simulink model "run_small_function_cov_bitadder"  (R2022b)
settings: Solver=VariableStepAuto  StartTime=0.0  StopTime=0.0  RelTol=1e-3
libraries: simulink x3193, hdlsllib x1590, ece1718_small_function x16
(part 25 of 26)

== system run_small_function_cov_bitadder/For Iterator Subsystem/train_top/batch/train_sub/conv_sig/filter dim iter /i ietar Subsystem/Subsystem/For Iterator Subsystem/mac/wt_multi/ca32/fa25 ==
  in1 : Inport  OutDataTypeStr=fixdt(0, 1, 0)  SampleTime=-1
  in2 : Inport  Port=2  OutDataTypeStr=fixdt(0, 1, 0)  SampleTime=-1
  Cin : Inport  Port=3  OutDataTypeStr=fixdt(0, 1, 0)  SampleTime=-1
  Bit_AND : simulink/Logic and Bit Operations/Bitwise Operator  logicop=AND  UseBitMask=off  NumInputPorts=2  BitMask=double(0)  BitMaskRealWorld=Real World Value
  Bit_AND_1 : simulink/Logic and Bit Operations/Bitwise Operator  logicop=AND  UseBitMask=off  NumInputPorts=2  BitMask=double(0)  BitMaskRealWorld=Real World Value
  Bit_OR : simulink/Logic and Bit Operations/Bitwise Operator  logicop=OR  UseBitMask=off  NumInputPorts=2  BitMask=double(0)  BitMaskRealWorld=Real World Value
  Bit_XOR : simulink/Logic and Bit Operations/Bitwise Operator  logicop=XOR  UseBitMask=off  NumInputPorts=2  BitMask=double(0)  BitMaskRealWorld=Real World Value
  Bit_XOR_1 : simulink/Logic and Bit Operations/Bitwise Operator  logicop=XOR  UseBitMask=off  NumInputPorts=2  BitMask=double(0)  BitMaskRealWorld=Real World Value
  Bit_XOR_2 : simulink/Logic and Bit Operations/Bitwise Operator  logicop=XOR  UseBitMask=off  NumInputPorts=2  BitMask=double(0)  BitMaskRealWorld=Real World Value
  S : Outport  OutDataTypeStr=fixdt(0, 1, 0)  SampleTime=-1
  C : Outport  Port=2  OutDataTypeStr=fixdt(0, 1, 0)  SampleTime=-1
  wires:
  in1/1 -> Bit_XOR_2/1, Bit_AND/1, Bit_XOR_1/1
  Cin/1 -> Bit_AND_1/1, Bit_XOR/2
  Bit_XOR/1 -> S/1
  Bit_AND/1 -> Bit_OR/1
  in2/1 -> Bit_XOR_2/2, Bit_AND/2, Bit_XOR_1/2
  Bit_AND_1/1 -> Bit_OR/2
  Bit_OR/1 -> C/1
  Bit_XOR_2/1 -> Bit_AND_1/2
  Bit_XOR_1/1 -> Bit_XOR/1

== system run_small_function_cov_bitadder/For Iterator Subsystem/train_top/batch/train_sub/conv_sig/filter dim iter /i ietar Subsystem/Subsystem/For Iterator Subsystem/mac/wt_multi/ca32/fa26 ==
  in1 : Inport  OutDataTypeStr=fixdt(0, 1, 0)  SampleTime=-1
  in2 : Inport  Port=2  OutDataTypeStr=fixdt(0, 1, 0)  SampleTime=-1
  Cin : Inport  Port=3  OutDataTypeStr=fixdt(0, 1, 0)  SampleTime=-1
  Bit_AND : simulink/Logic and Bit Operations/Bitwise Operator  logicop=AND  UseBitMask=off  NumInputPorts=2  BitMask=double(0)  BitMaskRealWorld=Real World Value
  Bit_AND_1 : simulink/Logic and Bit Operations/Bitwise Operator  logicop=AND  UseBitMask=off  NumInputPorts=2  BitMask=double(0)  BitMaskRealWorld=Real World Value
  Bit_OR : simulink/Logic and Bit Operations/Bitwise Operator  logicop=OR  UseBitMask=off  NumInputPorts=2  BitMask=double(0)  BitMaskRealWorld=Real World Value
  Bit_XOR : simulink/Logic and Bit Operations/Bitwise Operator  logicop=XOR  UseBitMask=off  NumInputPorts=2  BitMask=double(0)  BitMaskRealWorld=Real World Value
  Bit_XOR_1 : simulink/Logic and Bit Operations/Bitwise Operator  logicop=XOR  UseBitMask=off  NumInputPorts=2  BitMask=double(0)  BitMaskRealWorld=Real World Value
  Bit_XOR_2 : simulink/Logic and Bit Operations/Bitwise Operator  logicop=XOR  UseBitMask=off  NumInputPorts=2  BitMask=double(0)  BitMaskRealWorld=Real World Value
  S : Outport  OutDataTypeStr=fixdt(0, 1, 0)  SampleTime=-1
  C : Outport  Port=2  OutDataTypeStr=fixdt(0, 1, 0)  SampleTime=-1
  wires:
  in1/1 -> Bit_XOR_2/1, Bit_AND/1, Bit_XOR_1/1
  in2/1 -> Bit_XOR_2/2, Bit_AND/2, Bit_XOR_1/2
  Cin/1 -> Bit_AND_1/1, Bit_XOR/2
  Bit_AND_1/1 -> Bit_OR/2
  Bit_OR/1 -> C/1
  Bit_AND/1 -> Bit_OR/1
  Bit_XOR_2/1 -> Bit_AND_1/2
  Bit_XOR/1 -> S/1
  Bit_XOR_1/1 -> Bit_XOR/1

== system run_small_function_cov_bitadder/For Iterator Subsystem/train_top/batch/train_sub/conv_sig/filter dim iter /i ietar Subsystem/Subsystem/For Iterator Subsystem/mac/wt_multi/ca32/fa27 ==
  in1 : Inport  OutDataTypeStr=fixdt(0, 1, 0)  SampleTime=-1
  in2 : Inport  Port=2  OutDataTypeStr=fixdt(0, 1, 0)  SampleTime=-1
  Cin : Inport  Port=3  OutDataTypeStr=fixdt(0, 1, 0)  SampleTime=-1
  Bit_AND : simulink/Logic and Bit Operations/Bitwise Operator  logicop=AND  UseBitMask=off  NumInputPorts=2  BitMask=double(0)  BitMaskRealWorld=Real World Value
  Bit_AND_1 : simulink/Logic and Bit Operations/Bitwise Operator  logicop=AND  UseBitMask=off  NumInputPorts=2  BitMask=double(0)  BitMaskRealWorld=Real World Value
  Bit_OR : simulink/Logic and Bit Operations/Bitwise Operator  logicop=OR  UseBitMask=off  NumInputPorts=2  BitMask=double(0)  BitMaskRealWorld=Real World Value
  Bit_XOR : simulink/Logic and Bit Operations/Bitwise Operator  logicop=XOR  UseBitMask=off  NumInputPorts=2  BitMask=double(0)  BitMaskRealWorld=Real World Value
  Bit_XOR_1 : simulink/Logic and Bit Operations/Bitwise Operator  logicop=XOR  UseBitMask=off  NumInputPorts=2  BitMask=double(0)  BitMaskRealWorld=Real World Value
  Bit_XOR_2 : simulink/Logic and Bit Operations/Bitwise Operator  logicop=XOR  UseBitMask=off  NumInputPorts=2  BitMask=double(0)  BitMaskRealWorld=Real World Value
  S : Outport  OutDataTypeStr=fixdt(0, 1, 0)  SampleTime=-1
  C : Outport  Port=2  OutDataTypeStr=fixdt(0, 1, 0)  SampleTime=-1
  wires:
  in1/1 -> Bit_XOR_2/1, Bit_AND/1, Bit_XOR_1/1
  in2/1 -> Bit_XOR_2/2, Bit_AND/2, Bit_XOR_1/2
  Cin/1 -> Bit_AND_1/1, Bit_XOR/2
  Bit_AND_1/1 -> Bit_OR/2
  Bit_XOR/1 -> S/1
  Bit_OR/1 -> C/1
  Bit_XOR_2/1 -> Bit_AND_1/2
  Bit_AND/1 -> Bit_OR/1
  Bit_XOR_1/1 -> Bit_XOR/1

== system run_small_function_cov_bitadder/For Iterator Subsystem/train_top/batch/train_sub/conv_sig/filter dim iter /i ietar Subsystem/Subsystem/For Iterator Subsystem/mac/wt_multi/ca32/fa28 ==
  in1 : Inport  OutDataTypeStr=fixdt(0, 1, 0)  SampleTime=-1
  in2 : Inport  Port=2  OutDataTypeStr=fixdt(0, 1, 0)  SampleTime=-1
  Cin : Inport  Port=3  OutDataTypeStr=fixdt(0, 1, 0)  SampleTime=-1
  Bit_AND : simulink/Logic and Bit Operations/Bitwise Operator  logicop=AND  UseBitMask=off  NumInputPorts=2  BitMask=double(0)  BitMaskRealWorld=Real World Value
  Bit_AND_1 : simulink/Logic and Bit Operations/Bitwise Operator  logicop=AND  UseBitMask=off  NumInputPorts=2  BitMask=double(0)  BitMaskRealWorld=Real World Value
  Bit_OR : simulink/Logic and Bit Operations/Bitwise Operator  logicop=OR  UseBitMask=off  NumInputPorts=2  BitMask=double(0)  BitMaskRealWorld=Real World Value
  Bit_XOR : simulink/Logic and Bit Operations/Bitwise Operator  logicop=XOR  UseBitMask=off  NumInputPorts=2  BitMask=double(0)  BitMaskRealWorld=Real World Value
  Bit_XOR_1 : simulink/Logic and Bit Operations/Bitwise Operator  logicop=XOR  UseBitMask=off  NumInputPorts=2  BitMask=double(0)  BitMaskRealWorld=Real World Value
  Bit_XOR_2 : simulink/Logic and Bit Operations/Bitwise Operator  logicop=XOR  UseBitMask=off  NumInputPorts=2  BitMask=double(0)  BitMaskRealWorld=Real World Value
  S : Outport  OutDataTypeStr=fixdt(0, 1, 0)  SampleTime=-1
  C : Outport  Port=2  OutDataTypeStr=fixdt(0, 1, 0)  SampleTime=-1
  wires:
  in2/1 -> Bit_XOR_2/2, Bit_AND/2, Bit_XOR_1/2
  Bit_OR/1 -> C/1
  in1/1 -> Bit_XOR_2/1, Bit_AND/1, Bit_XOR_1/1
  Bit_AND/1 -> Bit_OR/1
  Bit_XOR/1 -> S/1
  Cin/1 -> Bit_AND_1/1, Bit_XOR/2
  Bit_AND_1/1 -> Bit_OR/2
  Bit_XOR_2/1 -> Bit_AND_1/2
  Bit_XOR_1/1 -> Bit_XOR/1

== system run_small_function_cov_bitadder/For Iterator Subsystem/train_top/batch/train_sub/conv_sig/filter dim iter /i ietar Subsystem/Subsystem/For Iterator Subsystem/mac/wt_multi/ca32/fa29 ==
  in1 : Inport  OutDataTypeStr=fixdt(0, 1, 0)  SampleTime=-1
  in2 : Inport  Port=2  OutDataTypeStr=fixdt(0, 1, 0)  SampleTime=-1
  Cin : Inport  Port=3  OutDataTypeStr=fixdt(0, 1, 0)  SampleTime=-1
  Bit_AND : simulink/Logic and Bit Operations/Bitwise Operator  logicop=AND  UseBitMask=off  NumInputPorts=2  BitMask=double(0)  BitMaskRealWorld=Real World Value
  Bit_AND_1 : simulink/Logic and Bit Operations/Bitwise Operator  logicop=AND  UseBitMask=off  NumInputPorts=2  BitMask=double(0)  BitMaskRealWorld=Real World Value
  Bit_OR : simulink/Logic and Bit Operations/Bitwise Operator  logicop=OR  UseBitMask=off  NumInputPorts=2  BitMask=double(0)  BitMaskRealWorld=Real World Value
  Bit_XOR : simulink/Logic and Bit Operations/Bitwise Operator  logicop=XOR  UseBitMask=off  NumInputPorts=2  BitMask=double(0)  BitMaskRealWorld=Real World Value
  Bit_XOR_1 : simulink/Logic and Bit Operations/Bitwise Operator  logicop=XOR  UseBitMask=off  NumInputPorts=2  BitMask=double(0)  BitMaskRealWorld=Real World Value
  Bit_XOR_2 : simulink/Logic and Bit Operations/Bitwise Operator  logicop=XOR  UseBitMask=off  NumInputPorts=2  BitMask=double(0)  BitMaskRealWorld=Real World Value
  S : Outport  OutDataTypeStr=fixdt(0, 1, 0)  SampleTime=-1
  C : Outport  Port=2  OutDataTypeStr=fixdt(0, 1, 0)  SampleTime=-1
  wires:
  in1/1 -> Bit_XOR_2/1, Bit_AND/1, Bit_XOR_1/1
  Cin/1 -> Bit_AND_1/1, Bit_XOR/2
  Bit_AND_1/1 -> Bit_OR/2
  Bit_OR/1 -> C/1
  Bit_XOR_2/1 -> Bit_AND_1/2
  Bit_XOR_1/1 -> Bit_XOR/1
  Bit_AND/1 -> Bit_OR/1
  in2/1 -> Bit_XOR_2/2, Bit_AND/2, Bit_XOR_1/2
  Bit_XOR/1 -> S/1

== system run_small_function_cov_bitadder/For Iterator Subsystem/train_top/batch/train_sub/conv_sig/filter dim iter /i ietar Subsystem/Subsystem/For Iterator Subsystem/mac/wt_multi/ca32/fa3 ==
  in1 : Inport  OutDataTypeStr=fixdt(0, 1, 0)  SampleTime=-1
  in2 : Inport  Port=2  OutDataTypeStr=fixdt(0, 1, 0)  SampleTime=-1
  Cin : Inport  Port=3  OutDataTypeStr=fixdt(0, 1, 0)  SampleTime=-1
  Bit_AND : simulink/Logic and Bit Operations/Bitwise Operator  logicop=AND  UseBitMask=off  NumInputPorts=2  BitMask=double(0)  BitMaskRealWorld=Real World Value
  Bit_AND_1 : simulink/Logic and Bit Operations/Bitwise Operator  logicop=AND  UseBitMask=off  NumInputPorts=2  BitMask=double(0)  BitMaskRealWorld=Real World Value
  Bit_OR : simulink/Logic and Bit Operations/Bitwise Operator  logicop=OR  UseBitMask=off  NumInputPorts=2  BitMask=double(0)  BitMaskRealWorld=Real World Value
  Bit_XOR : simulink/Logic and Bit Operations/Bitwise Operator  logicop=XOR  UseBitMask=off  NumInputPorts=2  BitMask=double(0)  BitMaskRealWorld=Real World Value
  Bit_XOR_1 : simulink/Logic and Bit Operations/Bitwise Operator  logicop=XOR  UseBitMask=off  NumInputPorts=2  BitMask=double(0)  BitMaskRealWorld=Real World Value
  Bit_XOR_2 : simulink/Logic and Bit Operations/Bitwise Operator  logicop=XOR  UseBitMask=off  NumInputPorts=2  BitMask=double(0)  BitMaskRealWorld=Real World Value
  S : Outport  OutDataTypeStr=fixdt(0, 1, 0)  SampleTime=-1
  C : Outport  Port=2  OutDataTypeStr=fixdt(0, 1, 0)  SampleTime=-1
  wires:
  in2/1 -> Bit_XOR_2/2, Bit_AND/2, Bit_XOR_1/2
  in1/1 -> Bit_XOR_2/1, Bit_AND/1, Bit_XOR_1/1
  Bit_AND_1/1 -> Bit_OR/2
  Bit_OR/1 -> C/1
  Cin/1 -> Bit_AND_1/1, Bit_XOR/2
  Bit_AND/1 -> Bit_OR/1
  Bit_XOR_2/1 -> Bit_AND_1/2
  Bit_XOR/1 -> S/1
  Bit_XOR_1/1 -> Bit_XOR/1

== system run_small_function_cov_bitadder/For Iterator Subsystem/train_top/batch/train_sub/conv_sig/filter dim iter /i ietar Subsystem/Subsystem/For Iterator Subsystem/mac/wt_multi/ca32/fa30 ==
  in1 : Inport  OutDataTypeStr=fixdt(0, 1, 0)  SampleTime=-1
  in2 : Inport  Port=2  OutDataTypeStr=fixdt(0, 1, 0)  SampleTime=-1
  Cin : Inport  Port=3  OutDataTypeStr=fixdt(0, 1, 0)  SampleTime=-1
  Bit_AND : simulink/Logic and Bit Operations/Bitwise Operator  logicop=AND  UseBitMask=off  NumInputPorts=2  BitMask=double(0)  BitMaskRealWorld=Real World Value
  Bit_AND_1 : simulink/Logic and Bit Operations/Bitwise Operator  logicop=AND  UseBitMask=off  NumInputPorts=2  BitMask=double(0)  BitMaskRealWorld=Real World Value
  Bit_OR : simulink/Logic and Bit Operations/Bitwise Operator  logicop=OR  UseBitMask=off  NumInputPorts=2  BitMask=double(0)  BitMaskRealWorld=Real World Value
  Bit_XOR : simulink/Logic and Bit Operations/Bitwise Operator  logicop=XOR  UseBitMask=off  NumInputPorts=2  BitMask=double(0)  BitMaskRealWorld=Real World Value
  Bit_XOR_1 : simulink/Logic and Bit Operations/Bitwise Operator  logicop=XOR  UseBitMask=off  NumInputPorts=2  BitMask=double(0)  BitMaskRealWorld=Real World Value
  Bit_XOR_2 : simulink/Logic and Bit Operations/Bitwise Operator  logicop=XOR  UseBitMask=off  NumInputPorts=2  BitMask=double(0)  BitMaskRealWorld=Real World Value
  S : Outport  OutDataTypeStr=fixdt(0, 1, 0)  SampleTime=-1
  C : Outport  Port=2  OutDataTypeStr=fixdt(0, 1, 0)  SampleTime=-1
  wires:
  in1/1 -> Bit_XOR_2/1, Bit_AND/1, Bit_XOR_1/1
  in2/1 -> Bit_XOR_2/2, Bit_AND/2, Bit_XOR_1/2
  Cin/1 -> Bit_AND_1/1, Bit_XOR/2
  Bit_AND_1/1 -> Bit_OR/2
  Bit_AND/1 -> Bit_OR/1
  Bit_OR/1 -> C/1
  Bit_XOR_2/1 -> Bit_AND_1/2
  Bit_XOR/1 -> S/1
  Bit_XOR_1/1 -> Bit_XOR/1

== system run_small_function_cov_bitadder/For Iterator Subsystem/train_top/batch/train_sub/conv_sig/filter dim iter /i ietar Subsystem/Subsystem/For Iterator Subsystem/mac/wt_multi/ca32/fa4 ==
  in1 : Inport  OutDataTypeStr=fixdt(0, 1, 0)  SampleTime=-1
  in2 : Inport  Port=2  OutDataTypeStr=fixdt(0, 1, 0)  SampleTime=-1
  Cin : Inport  Port=3  OutDataTypeStr=fixdt(0, 1, 0)  SampleTime=-1
  Bit_AND : simulink/Logic and Bit Operations/Bitwise Operator  logicop=AND  UseBitMask=off  NumInputPorts=2  BitMask=double(0)  BitMaskRealWorld=Real World Value
  Bit_AND_1 : simulink/Logic and Bit Operations/Bitwise Operator  logicop=AND  UseBitMask=off  NumInputPorts=2  BitMask=double(0)  BitMaskRealWorld=Real World Value
  Bit_OR : simulink/Logic and Bit Operations/Bitwise Operator  logicop=OR  UseBitMask=off  NumInputPorts=2  BitMask=double(0)  BitMaskRealWorld=Real World Value
  Bit_XOR : simulink/Logic and Bit Operations/Bitwise Operator  logicop=XOR  UseBitMask=off  NumInputPorts=2  BitMask=double(0)  BitMaskRealWorld=Real World Value
  Bit_XOR_1 : simulink/Logic and Bit Operations/Bitwise Operator  logicop=XOR  UseBitMask=off  NumInputPorts=2  BitMask=double(0)  BitMaskRealWorld=Real World Value
  Bit_XOR_2 : simulink/Logic and Bit Operations/Bitwise Operator  logicop=XOR  UseBitMask=off  NumInputPorts=2  BitMask=double(0)  BitMaskRealWorld=Real World Value
  S : Outport  OutDataTypeStr=fixdt(0, 1, 0)  SampleTime=-1
  C : Outport  Port=2  OutDataTypeStr=fixdt(0, 1, 0)  SampleTime=-1
  wires:
  in1/1 -> Bit_XOR_2/1, Bit_AND/1, Bit_XOR_1/1
  in2/1 -> Bit_XOR_2/2, Bit_AND/2, Bit_XOR_1/2
  Bit_AND_1/1 -> Bit_OR/2
  Cin/1 -> Bit_AND_1/1, Bit_XOR/2
  Bit_XOR_2/1 -> Bit_AND_1/2
  Bit_XOR_1/1 -> Bit_XOR/1
  Bit_OR/1 -> C/1
  Bit_XOR/1 -> S/1
  Bit_AND/1 -> Bit_OR/1

== system run_small_function_cov_bitadder/For Iterator Subsystem/train_top/batch/train_sub/conv_sig/filter dim iter /i ietar Subsystem/Subsystem/For Iterator Subsystem/mac/wt_multi/ca32/fa5 ==
  in1 : Inport  OutDataTypeStr=fixdt(0, 1, 0)  SampleTime=-1
  in2 : Inport  Port=2  OutDataTypeStr=fixdt(0, 1, 0)  SampleTime=-1
  Cin : Inport  Port=3  OutDataTypeStr=fixdt(0, 1, 0)  SampleTime=-1
  Bit_AND : simulink/Logic and Bit Operations/Bitwise Operator  logicop=AND  UseBitMask=off  NumInputPorts=2  BitMask=double(0)  BitMaskRealWorld=Real World Value
  Bit_AND_1 : simulink/Logic and Bit Operations/Bitwise Operator  logicop=AND  UseBitMask=off  NumInputPorts=2  BitMask=double(0)  BitMaskRealWorld=Real World Value
  Bit_OR : simulink/Logic and Bit Operations/Bitwise Operator  logicop=OR  UseBitMask=off  NumInputPorts=2  BitMask=double(0)  BitMaskRealWorld=Real World Value
  Bit_XOR : simulink/Logic and Bit Operations/Bitwise Operator  logicop=XOR  UseBitMask=off  NumInputPorts=2  BitMask=double(0)  BitMaskRealWorld=Real World Value
  Bit_XOR_1 : simulink/Logic and Bit Operations/Bitwise Operator  logicop=XOR  UseBitMask=off  NumInputPorts=2  BitMask=double(0)  BitMaskRealWorld=Real World Value
  Bit_XOR_2 : simulink/Logic and Bit Operations/Bitwise Operator  logicop=XOR  UseBitMask=off  NumInputPorts=2  BitMask=double(0)  BitMaskRealWorld=Real World Value
  S : Outport  OutDataTypeStr=fixdt(0, 1, 0)  SampleTime=-1
  C : Outport  Port=2  OutDataTypeStr=fixdt(0, 1, 0)  SampleTime=-1
  wires:
  in1/1 -> Bit_XOR_2/1, Bit_AND/1, Bit_XOR_1/1
  in2/1 -> Bit_XOR_2/2, Bit_AND/2, Bit_XOR_1/2
  Cin/1 -> Bit_AND_1/1, Bit_XOR/2
  Bit_AND_1/1 -> Bit_OR/2
  Bit_OR/1 -> C/1
  Bit_XOR_2/1 -> Bit_AND_1/2
  Bit_AND/1 -> Bit_OR/1
  Bit_XOR_1/1 -> Bit_XOR/1
  Bit_XOR/1 -> S/1

== system run_small_function_cov_bitadder/For Iterator Subsystem/train_top/batch/train_sub/conv_sig/filter dim iter /i ietar Subsystem/Subsystem/For Iterator Subsystem/mac/wt_multi/ca32/fa6 ==
  in1 : Inport  OutDataTypeStr=fixdt(0, 1, 0)  SampleTime=-1
  in2 : Inport  Port=2  OutDataTypeStr=fixdt(0, 1, 0)  SampleTime=-1
  Cin : Inport  Port=3  OutDataTypeStr=fixdt(0, 1, 0)  SampleTime=-1
  Bit_AND : simulink/Logic and Bit Operations/Bitwise Operator  logicop=AND  UseBitMask=off  NumInputPorts=2  BitMask=double(0)  BitMaskRealWorld=Real World Value
  Bit_AND_1 : simulink/Logic and Bit Operations/Bitwise Operator  logicop=AND  UseBitMask=off  NumInputPorts=2  BitMask=double(0)  BitMaskRealWorld=Real World Value
  Bit_OR : simulink/Logic and Bit Operations/Bitwise Operator  logicop=OR  UseBitMask=off  NumInputPorts=2  BitMask=double(0)  BitMaskRealWorld=Real World Value
  Bit_XOR : simulink/Logic and Bit Operations/Bitwise Operator  logicop=XOR  UseBitMask=off  NumInputPorts=2  BitMask=double(0)  BitMaskRealWorld=Real World Value
  Bit_XOR_1 : simulink/Logic and Bit Operations/Bitwise Operator  logicop=XOR  UseBitMask=off  NumInputPorts=2  BitMask=double(0)  BitMaskRealWorld=Real World Value
  Bit_XOR_2 : simulink/Logic and Bit Operations/Bitwise Operator  logicop=XOR  UseBitMask=off  NumInputPorts=2  BitMask=double(0)  BitMaskRealWorld=Real World Value
  S : Outport  OutDataTypeStr=fixdt(0, 1, 0)  SampleTime=-1
  C : Outport  Port=2  OutDataTypeStr=fixdt(0, 1, 0)  SampleTime=-1
  wires:
  in1/1 -> Bit_XOR_2/1, Bit_AND/1, Bit_XOR_1/1
  in2/1 -> Bit_XOR_2/2, Bit_AND/2, Bit_XOR_1/2
  Bit_AND_1/1 -> Bit_OR/2
  Bit_OR/1 -> C/1
  Bit_XOR/1 -> S/1
  Bit_XOR_2/1 -> Bit_AND_1/2
  Cin/1 -> Bit_AND_1/1, Bit_XOR/2
  Bit_AND/1 -> Bit_OR/1
  Bit_XOR_1/1 -> Bit_XOR/1

== system run_small_function_cov_bitadder/For Iterator Subsystem/train_top/batch/train_sub/conv_sig/filter dim iter /i ietar Subsystem/Subsystem/For Iterator Subsystem/mac/wt_multi/ca32/fa7 ==
  in1 : Inport  OutDataTypeStr=fixdt(0, 1, 0)  SampleTime=-1
  in2 : Inport  Port=2  OutDataTypeStr=fixdt(0, 1, 0)  SampleTime=-1
  Cin : Inport  Port=3  OutDataTypeStr=fixdt(0, 1, 0)  SampleTime=-1
  Bit_AND : simulink/Logic and Bit Operations/Bitwise Operator  logicop=AND  UseBitMask=off  NumInputPorts=2  BitMask=double(0)  BitMaskRealWorld=Real World Value
  Bit_AND_1 : simulink/Logic and Bit Operations/Bitwise Operator  logicop=AND  UseBitMask=off  NumInputPorts=2  BitMask=double(0)  BitMaskRealWorld=Real World Value
  Bit_OR : simulink/Logic and Bit Operations/Bitwise Operator  logicop=OR  UseBitMask=off  NumInputPorts=2  BitMask=double(0)  BitMaskRealWorld=Real World Value
  Bit_XOR : simulink/Logic and Bit Operations/Bitwise Operator  logicop=XOR  UseBitMask=off  NumInputPorts=2  BitMask=double(0)  BitMaskRealWorld=Real World Value
  Bit_XOR_1 : simulink/Logic and Bit Operations/Bitwise Operator  logicop=XOR  UseBitMask=off  NumInputPorts=2  BitMask=double(0)  BitMaskRealWorld=Real World Value
  Bit_XOR_2 : simulink/Logic and Bit Operations/Bitwise Operator  logicop=XOR  UseBitMask=off  NumInputPorts=2  BitMask=double(0)  BitMaskRealWorld=Real World Value
  S : Outport  OutDataTypeStr=fixdt(0, 1, 0)  SampleTime=-1
  C : Outport  Port=2  OutDataTypeStr=fixdt(0, 1, 0)  SampleTime=-1
  wires:
  in1/1 -> Bit_XOR_2/1, Bit_AND/1, Bit_XOR_1/1
  in2/1 -> Bit_XOR_2/2, Bit_AND/2, Bit_XOR_1/2
  Cin/1 -> Bit_AND_1/1, Bit_XOR/2
  Bit_OR/1 -> C/1
  Bit_XOR_2/1 -> Bit_AND_1/2
  Bit_AND_1/1 -> Bit_OR/2
  Bit_XOR/1 -> S/1
  Bit_AND/1 -> Bit_OR/1
  Bit_XOR_1/1 -> Bit_XOR/1

== system run_small_function_cov_bitadder/For Iterator Subsystem/train_top/batch/train_sub/conv_sig/filter dim iter /i ietar Subsystem/Subsystem/For Iterator Subsystem/mac/wt_multi/ca32/fa8 ==
  in1 : Inport  OutDataTypeStr=fixdt(0, 1, 0)  SampleTime=-1
  in2 : Inport  Port=2  OutDataTypeStr=fixdt(0, 1, 0)  SampleTime=-1
  Cin : Inport  Port=3  OutDataTypeStr=fixdt(0, 1, 0)  SampleTime=-1
  Bit_AND : simulink/Logic and Bit Operations/Bitwise Operator  logicop=AND  UseBitMask=off  NumInputPorts=2  BitMask=double(0)  BitMaskRealWorld=Real World Value
  Bit_AND_1 : simulink/Logic and Bit Operations/Bitwise Operator  logicop=AND  UseBitMask=off  NumInputPorts=2  BitMask=double(0)  BitMaskRealWorld=Real World Value
  Bit_OR : simulink/Logic and Bit Operations/Bitwise Operator  logicop=OR  UseBitMask=off  NumInputPorts=2  BitMask=double(0)  BitMaskRealWorld=Real World Value
  Bit_XOR : simulink/Logic and Bit Operations/Bitwise Operator  logicop=XOR  UseBitMask=off  NumInputPorts=2  BitMask=double(0)  BitMaskRealWorld=Real World Value
  Bit_XOR_1 : simulink/Logic and Bit Operations/Bitwise Operator  logicop=XOR  UseBitMask=off  NumInputPorts=2  BitMask=double(0)  BitMaskRealWorld=Real World Value
  Bit_XOR_2 : simulink/Logic and Bit Operations/Bitwise Operator  logicop=XOR  UseBitMask=off  NumInputPorts=2  BitMask=double(0)  BitMaskRealWorld=Real World Value
  S : Outport  OutDataTypeStr=fixdt(0, 1, 0)  SampleTime=-1
  C : Outport  Port=2  OutDataTypeStr=fixdt(0, 1, 0)  SampleTime=-1
  wires:
  in1/1 -> Bit_XOR_2/1, Bit_AND/1, Bit_XOR_1/1
  in2/1 -> Bit_XOR_2/2, Bit_AND/2, Bit_XOR_1/2
  Cin/1 -> Bit_AND_1/1, Bit_XOR/2
  Bit_AND_1/1 -> Bit_OR/2
  Bit_OR/1 -> C/1
  Bit_XOR_2/1 -> Bit_AND_1/2
  Bit_XOR/1 -> S/1
  Bit_AND/1 -> Bit_OR/1
  Bit_XOR_1/1 -> Bit_XOR/1

== system run_small_function_cov_bitadder/For Iterator Subsystem/train_top/batch/train_sub/conv_sig/filter dim iter /i ietar Subsystem/Subsystem/For Iterator Subsystem/mac/wt_multi/ca32/fa9 ==
  in1 : Inport  OutDataTypeStr=fixdt(0, 1, 0)  SampleTime=-1
  in2 : Inport  Port=2  OutDataTypeStr=fixdt(0, 1, 0)  SampleTime=-1
  Cin : Inport  Port=3  OutDataTypeStr=fixdt(0, 1, 0)  SampleTime=-1
  Bit_AND : simulink/Logic and Bit Operations/Bitwise Operator  logicop=AND  UseBitMask=off  NumInputPorts=2  BitMask=double(0)  BitMaskRealWorld=Real World Value
  Bit_AND_1 : simulink/Logic and Bit Operations/Bitwise Operator  logicop=AND  UseBitMask=off  NumInputPorts=2  BitMask=double(0)  BitMaskRealWorld=Real World Value
  Bit_OR : simulink/Logic and Bit Operations/Bitwise Operator  logicop=OR  UseBitMask=off  NumInputPorts=2  BitMask=double(0)  BitMaskRealWorld=Real World Value
  Bit_XOR : simulink/Logic and Bit Operations/Bitwise Operator  logicop=XOR  UseBitMask=off  NumInputPorts=2  BitMask=double(0)  BitMaskRealWorld=Real World Value
  Bit_XOR_1 : simulink/Logic and Bit Operations/Bitwise Operator  logicop=XOR  UseBitMask=off  NumInputPorts=2  BitMask=double(0)  BitMaskRealWorld=Real World Value
  Bit_XOR_2 : simulink/Logic and Bit Operations/Bitwise Operator  logicop=XOR  UseBitMask=off  NumInputPorts=2  BitMask=double(0)  BitMaskRealWorld=Real World Value
  S : Outport  OutDataTypeStr=fixdt(0, 1, 0)  SampleTime=-1
  C : Outport  Port=2  OutDataTypeStr=fixdt(0, 1, 0)  SampleTime=-1
  wires:
  in1/1 -> Bit_XOR_2/1, Bit_AND/1, Bit_XOR_1/1
  in2/1 -> Bit_XOR_2/2, Bit_AND/2, Bit_XOR_1/2
  Cin/1 -> Bit_AND_1/1, Bit_XOR/2
  Bit_AND_1/1 -> Bit_OR/2
  Bit_OR/1 -> C/1
  Bit_XOR/1 -> S/1
  Bit_XOR_2/1 -> Bit_AND_1/2
  Bit_XOR_1/1 -> Bit_XOR/1
  Bit_AND/1 -> Bit_OR/1

== system run_small_function_cov_bitadder/For Iterator Subsystem/train_top/batch/train_sub/conv_sig/filter dim iter /i ietar Subsystem/Subsystem/For Iterator Subsystem/mac/wt_multi/ra/fa0 ==
  in1 : Inport  OutDataTypeStr=fixdt(0, 1, 0)  SampleTime=-1
  in2 : Inport  Port=2  OutDataTypeStr=fixdt(0, 1, 0)  SampleTime=-1
  Cin : Inport  Port=3  OutDataTypeStr=fixdt(0, 1, 0)  SampleTime=-1
  Bit_AND : simulink/Logic and Bit Operations/Bitwise Operator  logicop=AND  UseBitMask=off  NumInputPorts=2  BitMask=double(0)  BitMaskRealWorld=Real World Value
  Bit_AND_1 : simulink/Logic and Bit Operations/Bitwise Operator  logicop=AND  UseBitMask=off  NumInputPorts=2  BitMask=double(0)  BitMaskRealWorld=Real World Value
  Bit_OR : simulink/Logic and Bit Operations/Bitwise Operator  logicop=OR  UseBitMask=off  NumInputPorts=2  BitMask=double(0)  BitMaskRealWorld=Real World Value
  Bit_XOR : simulink/Logic and Bit Operations/Bitwise Operator  logicop=XOR  UseBitMask=off  NumInputPorts=2  BitMask=double(0)  BitMaskRealWorld=Real World Value
  Bit_XOR_1 : simulink/Logic and Bit Operations/Bitwise Operator  logicop=XOR  UseBitMask=off  NumInputPorts=2  BitMask=double(0)  BitMaskRealWorld=Real World Value
  Bit_XOR_2 : simulink/Logic and Bit Operations/Bitwise Operator  logicop=XOR  UseBitMask=off  NumInputPorts=2  BitMask=double(0)  BitMaskRealWorld=Real World Value
  S : Outport  OutDataTypeStr=fixdt(0, 1, 0)  SampleTime=-1
  C : Outport  Port=2  OutDataTypeStr=fixdt(0, 1, 0)  SampleTime=-1
  wires:
  in1/1 -> Bit_XOR_2/1, Bit_AND/1, Bit_XOR_1/1
  Cin/1 -> Bit_AND_1/1, Bit_XOR/2
  Bit_AND_1/1 -> Bit_OR/2
  Bit_OR/1 -> C/1
  Bit_XOR_2/1 -> Bit_AND_1/2
  Bit_XOR/1 -> S/1
  in2/1 -> Bit_XOR_2/2, Bit_AND/2, Bit_XOR_1/2
  Bit_AND/1 -> Bit_OR/1
  Bit_XOR_1/1 -> Bit_XOR/1

== system run_small_function_cov_bitadder/For Iterator Subsystem/train_top/batch/train_sub/conv_sig/filter dim iter /i ietar Subsystem/Subsystem/For Iterator Subsystem/mac/wt_multi/ra/fa1 ==
  in1 : Inport  OutDataTypeStr=fixdt(0, 1, 0)  SampleTime=-1
  in2 : Inport  Port=2  OutDataTypeStr=fixdt(0, 1, 0)  SampleTime=-1
  Cin : Inport  Port=3  OutDataTypeStr=fixdt(0, 1, 0)  SampleTime=-1
  Bit_AND : simulink/Logic and Bit Operations/Bitwise Operator  logicop=AND  UseBitMask=off  NumInputPorts=2  BitMask=double(0)  BitMaskRealWorld=Real World Value
  Bit_AND_1 : simulink/Logic and Bit Operations/Bitwise Operator  logicop=AND  UseBitMask=off  NumInputPorts=2  BitMask=double(0)  BitMaskRealWorld=Real World Value
  Bit_OR : simulink/Logic and Bit Operations/Bitwise Operator  logicop=OR  UseBitMask=off  NumInputPorts=2  BitMask=double(0)  BitMaskRealWorld=Real World Value
  Bit_XOR : simulink/Logic and Bit Operations/Bitwise Operator  logicop=XOR  UseBitMask=off  NumInputPorts=2  BitMask=double(0)  BitMaskRealWorld=Real World Value
  Bit_XOR_1 : simulink/Logic and Bit Operations/Bitwise Operator  logicop=XOR  UseBitMask=off  NumInputPorts=2  BitMask=double(0)  BitMaskRealWorld=Real World Value
  Bit_XOR_2 : simulink/Logic and Bit Operations/Bitwise Operator  logicop=XOR  UseBitMask=off  NumInputPorts=2  BitMask=double(0)  BitMaskRealWorld=Real World Value
  S : Outport  OutDataTypeStr=fixdt(0, 1, 0)  SampleTime=-1
  C : Outport  Port=2  OutDataTypeStr=fixdt(0, 1, 0)  SampleTime=-1
  wires:
  in1/1 -> Bit_XOR_2/1, Bit_AND/1, Bit_XOR_1/1
  in2/1 -> Bit_XOR_2/2, Bit_AND/2, Bit_XOR_1/2
  Cin/1 -> Bit_AND_1/1, Bit_XOR/2
  Bit_AND_1/1 -> Bit_OR/2
  Bit_OR/1 -> C/1
  Bit_XOR/1 -> S/1
  Bit_XOR_1/1 -> Bit_XOR/1
  Bit_AND/1 -> Bit_OR/1
  Bit_XOR_2/1 -> Bit_AND_1/2

== system run_small_function_cov_bitadder/For Iterator Subsystem/train_top/batch/train_sub/conv_sig/filter dim iter /i ietar Subsystem/Subsystem/For Iterator Subsystem/mac/wt_multi/ra/fa10 ==
  in1 : Inport  OutDataTypeStr=fixdt(0, 1, 0)  SampleTime=-1
  in2 : Inport  Port=2  OutDataTypeStr=fixdt(0, 1, 0)  SampleTime=-1
  Cin : Inport  Port=3  OutDataTypeStr=fixdt(0, 1, 0)  SampleTime=-1
  Bit_AND : simulink/Logic and Bit Operations/Bitwise Operator  logicop=AND  UseBitMask=off  NumInputPorts=2  BitMask=double(0)  BitMaskRealWorld=Real World Value
  Bit_AND_1 : simulink/Logic and Bit Operations/Bitwise Operator  logicop=AND  UseBitMask=off  NumInputPorts=2  BitMask=double(0)  BitMaskRealWorld=Real World Value
  Bit_OR : simulink/Logic and Bit Operations/Bitwise Operator  logicop=OR  UseBitMask=off  NumInputPorts=2  BitMask=double(0)  BitMaskRealWorld=Real World Value
  Bit_XOR : simulink/Logic and Bit Operations/Bitwise Operator  logicop=XOR  UseBitMask=off  NumInputPorts=2  BitMask=double(0)  BitMaskRealWorld=Real World Value
  Bit_XOR_1 : simulink/Logic and Bit Operations/Bitwise Operator  logicop=XOR  UseBitMask=off  NumInputPorts=2  BitMask=double(0)  BitMaskRealWorld=Real World Value
  Bit_XOR_2 : simulink/Logic and Bit Operations/Bitwise Operator  logicop=XOR  UseBitMask=off  NumInputPorts=2  BitMask=double(0)  BitMaskRealWorld=Real World Value
  S : Outport  OutDataTypeStr=fixdt(0, 1, 0)  SampleTime=-1
  C : Outport  Port=2  OutDataTypeStr=fixdt(0, 1, 0)  SampleTime=-1
  wires:
  in1/1 -> Bit_XOR_2/1, Bit_AND/1, Bit_XOR_1/1
  Cin/1 -> Bit_AND_1/1, Bit_XOR/2
  Bit_AND_1/1 -> Bit_OR/2
  Bit_OR/1 -> C/1
  in2/1 -> Bit_XOR_2/2, Bit_AND/2, Bit_XOR_1/2
  Bit_XOR_2/1 -> Bit_AND_1/2
  Bit_XOR_1/1 -> Bit_XOR/1
  Bit_AND/1 -> Bit_OR/1
  Bit_XOR/1 -> S/1

== system run_small_function_cov_bitadder/For Iterator Subsystem/train_top/batch/train_sub/conv_sig/filter dim iter /i ietar Subsystem/Subsystem/For Iterator Subsystem/mac/wt_multi/ra/fa11 ==
  in1 : Inport  OutDataTypeStr=fixdt(0, 1, 0)  SampleTime=-1
  in2 : Inport  Port=2  OutDataTypeStr=fixdt(0, 1, 0)  SampleTime=-1
  Cin : Inport  Port=3  OutDataTypeStr=fixdt(0, 1, 0)  SampleTime=-1
  Bit_AND : simulink/Logic and Bit Operations/Bitwise Operator  logicop=AND  UseBitMask=off  NumInputPorts=2  BitMask=double(0)  BitMaskRealWorld=Real World Value
  Bit_AND_1 : simulink/Logic and Bit Operations/Bitwise Operator  logicop=AND  UseBitMask=off  NumInputPorts=2  BitMask=double(0)  BitMaskRealWorld=Real World Value
  Bit_OR : simulink/Logic and Bit Operations/Bitwise Operator  logicop=OR  UseBitMask=off  NumInputPorts=2  BitMask=double(0)  BitMaskRealWorld=Real World Value
  Bit_XOR : simulink/Logic and Bit Operations/Bitwise Operator  logicop=XOR  UseBitMask=off  NumInputPorts=2  BitMask=double(0)  BitMaskRealWorld=Real World Value
  Bit_XOR_1 : simulink/Logic and Bit Operations/Bitwise Operator  logicop=XOR  UseBitMask=off  NumInputPorts=2  BitMask=double(0)  BitMaskRealWorld=Real World Value
  Bit_XOR_2 : simulink/Logic and Bit Operations/Bitwise Operator  logicop=XOR  UseBitMask=off  NumInputPorts=2  BitMask=double(0)  BitMaskRealWorld=Real World Value
  S : Outport  OutDataTypeStr=fixdt(0, 1, 0)  SampleTime=-1
  C : Outport  Port=2  OutDataTypeStr=fixdt(0, 1, 0)  SampleTime=-1
  wires:
  in2/1 -> Bit_XOR_2/2, Bit_AND/2, Bit_XOR_1/2
  Cin/1 -> Bit_AND_1/1, Bit_XOR/2
  Bit_AND_1/1 -> Bit_OR/2
  in1/1 -> Bit_XOR_2/1, Bit_AND/1, Bit_XOR_1/1
  Bit_OR/1 -> C/1
  Bit_XOR/1 -> S/1
  Bit_XOR_2/1 -> Bit_AND_1/2
  Bit_AND/1 -> Bit_OR/1
  Bit_XOR_1/1 -> Bit_XOR/1

== system run_small_function_cov_bitadder/For Iterator Subsystem/train_top/batch/train_sub/conv_sig/filter dim iter /i ietar Subsystem/Subsystem/For Iterator Subsystem/mac/wt_multi/ra/fa12 ==
  in1 : Inport  OutDataTypeStr=fixdt(0, 1, 0)  SampleTime=-1
  in2 : Inport  Port=2  OutDataTypeStr=fixdt(0, 1, 0)  SampleTime=-1
  Cin : Inport  Port=3  OutDataTypeStr=fixdt(0, 1, 0)  SampleTime=-1
  Bit_AND : simulink/Logic and Bit Operations/Bitwise Operator  logicop=AND  UseBitMask=off  NumInputPorts=2  BitMask=double(0)  BitMaskRealWorld=Real World Value
  Bit_AND_1 : simulink/Logic and Bit Operations/Bitwise Operator  logicop=AND  UseBitMask=off  NumInputPorts=2  BitMask=double(0)  BitMaskRealWorld=Real World Value
  Bit_OR : simulink/Logic and Bit Operations/Bitwise Operator  logicop=OR  UseBitMask=off  NumInputPorts=2  BitMask=double(0)  BitMaskRealWorld=Real World Value
  Bit_XOR : simulink/Logic and Bit Operations/Bitwise Operator  logicop=XOR  UseBitMask=off  NumInputPorts=2  BitMask=double(0)  BitMaskRealWorld=Real World Value
  Bit_XOR_1 : simulink/Logic and Bit Operations/Bitwise Operator  logicop=XOR  UseBitMask=off  NumInputPorts=2  BitMask=double(0)  BitMaskRealWorld=Real World Value
  Bit_XOR_2 : simulink/Logic and Bit Operations/Bitwise Operator  logicop=XOR  UseBitMask=off  NumInputPorts=2  BitMask=double(0)  BitMaskRealWorld=Real World Value
  S : Outport  OutDataTypeStr=fixdt(0, 1, 0)  SampleTime=-1
  C : Outport  Port=2  OutDataTypeStr=fixdt(0, 1, 0)  SampleTime=-1
  wires:
  in2/1 -> Bit_XOR_2/2, Bit_AND/2, Bit_XOR_1/2
  Cin/1 -> Bit_AND_1/1, Bit_XOR/2
  in1/1 -> Bit_XOR_2/1, Bit_AND/1, Bit_XOR_1/1
  Bit_OR/1 -> C/1
  Bit_XOR_2/1 -> Bit_AND_1/2
  Bit_AND_1/1 -> Bit_OR/2
  Bit_AND/1 -> Bit_OR/1
  Bit_XOR/1 -> S/1
  Bit_XOR_1/1 -> Bit_XOR/1

== system run_small_function_cov_bitadder/For Iterator Subsystem/train_top/batch/train_sub/conv_sig/filter dim iter /i ietar Subsystem/Subsystem/For Iterator Subsystem/mac/wt_multi/ra/fa13 ==
  in1 : Inport  OutDataTypeStr=fixdt(0, 1, 0)  SampleTime=-1
  in2 : Inport  Port=2  OutDataTypeStr=fixdt(0, 1, 0)  SampleTime=-1
  Cin : Inport  Port=3  OutDataTypeStr=fixdt(0, 1, 0)  SampleTime=-1
  Bit_AND : simulink/Logic and Bit Operations/Bitwise Operator  logicop=AND  UseBitMask=off  NumInputPorts=2  BitMask=double(0)  BitMaskRealWorld=Real World Value
  Bit_AND_1 : simulink/Logic and Bit Operations/Bitwise Operator  logicop=AND  UseBitMask=off  NumInputPorts=2  BitMask=double(0)  BitMaskRealWorld=Real World Value
  Bit_OR : simulink/Logic and Bit Operations/Bitwise Operator  logicop=OR  UseBitMask=off  NumInputPorts=2  BitMask=double(0)  BitMaskRealWorld=Real World Value
  Bit_XOR : simulink/Logic and Bit Operations/Bitwise Operator  logicop=XOR  UseBitMask=off  NumInputPorts=2  BitMask=double(0)  BitMaskRealWorld=Real World Value
  Bit_XOR_1 : simulink/Logic and Bit Operations/Bitwise Operator  logicop=XOR  UseBitMask=off  NumInputPorts=2  BitMask=double(0)  BitMaskRealWorld=Real World Value
  Bit_XOR_2 : simulink/Logic and Bit Operations/Bitwise Operator  logicop=XOR  UseBitMask=off  NumInputPorts=2  BitMask=double(0)  BitMaskRealWorld=Real World Value
  S : Outport  OutDataTypeStr=fixdt(0, 1, 0)  SampleTime=-1
  C : Outport  Port=2  OutDataTypeStr=fixdt(0, 1, 0)  SampleTime=-1
  wires:
  in1/1 -> Bit_XOR_2/1, Bit_AND/1, Bit_XOR_1/1
  in2/1 -> Bit_XOR_2/2, Bit_AND/2, Bit_XOR_1/2
  Cin/1 -> Bit_AND_1/1, Bit_XOR/2
  Bit_AND_1/1 -> Bit_OR/2
  Bit_OR/1 -> C/1
  Bit_XOR_2/1 -> Bit_AND_1/2
  Bit_AND/1 -> Bit_OR/1
  Bit_XOR/1 -> S/1
  Bit_XOR_1/1 -> Bit_XOR/1

== system run_small_function_cov_bitadder/For Iterator Subsystem/train_top/batch/train_sub/conv_sig/filter dim iter /i ietar Subsystem/Subsystem/For Iterator Subsystem/mac/wt_multi/ra/fa14 ==
  in1 : Inport  OutDataTypeStr=fixdt(0, 1, 0)  SampleTime=-1
  in2 : Inport  Port=2  OutDataTypeStr=fixdt(0, 1, 0)  SampleTime=-1
  Cin : Inport  Port=3  OutDataTypeStr=fixdt(0, 1, 0)  SampleTime=-1
  Bit_AND : simulink/Logic and Bit Operations/Bitwise Operator  logicop=AND  UseBitMask=off  NumInputPorts=2  BitMask=double(0)  BitMaskRealWorld=Real World Value
  Bit_AND_1 : simulink/Logic and Bit Operations/Bitwise Operator  logicop=AND  UseBitMask=off  NumInputPorts=2  BitMask=double(0)  BitMaskRealWorld=Real World Value
  Bit_OR : simulink/Logic and Bit Operations/Bitwise Operator  logicop=OR  UseBitMask=off  NumInputPorts=2  BitMask=double(0)  BitMaskRealWorld=Real World Value
  Bit_XOR : simulink/Logic and Bit Operations/Bitwise Operator  logicop=XOR  UseBitMask=off  NumInputPorts=2  BitMask=double(0)  BitMaskRealWorld=Real World Value
  Bit_XOR_1 : simulink/Logic and Bit Operations/Bitwise Operator  logicop=XOR  UseBitMask=off  NumInputPorts=2  BitMask=double(0)  BitMaskRealWorld=Real World Value
  Bit_XOR_2 : simulink/Logic and Bit Operations/Bitwise Operator  logicop=XOR  UseBitMask=off  NumInputPorts=2  BitMask=double(0)  BitMaskRealWorld=Real World Value
  S : Outport  OutDataTypeStr=fixdt(0, 1, 0)  SampleTime=-1
  C : Outport  Port=2  OutDataTypeStr=fixdt(0, 1, 0)  SampleTime=-1
  wires:
  in1/1 -> Bit_XOR_2/1, Bit_AND/1, Bit_XOR_1/1
  Cin/1 -> Bit_AND_1/1, Bit_XOR/2
  Bit_AND_1/1 -> Bit_OR/2
  Bit_XOR_2/1 -> Bit_AND_1/2
  in2/1 -> Bit_XOR_2/2, Bit_AND/2, Bit_XOR_1/2
  Bit_OR/1 -> C/1
  Bit_AND/1 -> Bit_OR/1
  Bit_XOR/1 -> S/1
  Bit_XOR_1/1 -> Bit_XOR/1

== system run_small_function_cov_bitadder/For Iterator Subsystem/train_top/batch/train_sub/conv_sig/filter dim iter /i ietar Subsystem/Subsystem/For Iterator Subsystem/mac/wt_multi/ra/fa15 ==
  in1 : Inport  OutDataTypeStr=fixdt(0, 1, 0)  SampleTime=-1
  in2 : Inport  Port=2  OutDataTypeStr=fixdt(0, 1, 0)  SampleTime=-1
  Cin : Inport  Port=3  OutDataTypeStr=fixdt(0, 1, 0)  SampleTime=-1
  Bit_AND : simulink/Logic and Bit Operations/Bitwise Operator  logicop=AND  UseBitMask=off  NumInputPorts=2  BitMask=double(0)  BitMaskRealWorld=Real World Value
  Bit_AND_1 : simulink/Logic and Bit Operations/Bitwise Operator  logicop=AND  UseBitMask=off  NumInputPorts=2  BitMask=double(0)  BitMaskRealWorld=Real World Value
  Bit_OR : simulink/Logic and Bit Operations/Bitwise Operator  logicop=OR  UseBitMask=off  NumInputPorts=2  BitMask=double(0)  BitMaskRealWorld=Real World Value
  Bit_XOR : simulink/Logic and Bit Operations/Bitwise Operator  logicop=XOR  UseBitMask=off  NumInputPorts=2  BitMask=double(0)  BitMaskRealWorld=Real World Value
  Bit_XOR_1 : simulink/Logic and Bit Operations/Bitwise Operator  logicop=XOR  UseBitMask=off  NumInputPorts=2  BitMask=double(0)  BitMaskRealWorld=Real World Value
  Bit_XOR_2 : simulink/Logic and Bit Operations/Bitwise Operator  logicop=XOR  UseBitMask=off  NumInputPorts=2  BitMask=double(0)  BitMaskRealWorld=Real World Value
  S : Outport  OutDataTypeStr=fixdt(0, 1, 0)  SampleTime=-1
  C : Outport  Port=2  OutDataTypeStr=fixdt(0, 1, 0)  SampleTime=-1
  wires:
  in1/1 -> Bit_XOR_2/1, Bit_AND/1, Bit_XOR_1/1
  in2/1 -> Bit_XOR_2/2, Bit_AND/2, Bit_XOR_1/2
  Cin/1 -> Bit_AND_1/1, Bit_XOR/2
  Bit_AND_1/1 -> Bit_OR/2
  Bit_OR/1 -> C/1
  Bit_XOR_2/1 -> Bit_AND_1/2
  Bit_AND/1 -> Bit_OR/1
  Bit_XOR_1/1 -> Bit_XOR/1
  Bit_XOR/1 -> S/1

== system run_small_function_cov_bitadder/For Iterator Subsystem/train_top/batch/train_sub/conv_sig/filter dim iter /i ietar Subsystem/Subsystem/For Iterator Subsystem/mac/wt_multi/ra/fa16 ==
  in1 : Inport  OutDataTypeStr=fixdt(0, 1, 0)  SampleTime=-1
  in2 : Inport  Port=2  OutDataTypeStr=fixdt(0, 1, 0)  SampleTime=-1
  Cin : Inport  Port=3  OutDataTypeStr=fixdt(0, 1, 0)  SampleTime=-1
  Bit_AND : simulink/Logic and Bit Operations/Bitwise Operator  logicop=AND  UseBitMask=off  NumInputPorts=2  BitMask=double(0)  BitMaskRealWorld=Real World Value
  Bit_AND_1 : simulink/Logic and Bit Operations/Bitwise Operator  logicop=AND  UseBitMask=off  NumInputPorts=2  BitMask=double(0)  BitMaskRealWorld=Real World Value
  Bit_OR : simulink/Logic and Bit Operations/Bitwise Operator  logicop=OR  UseBitMask=off  NumInputPorts=2  BitMask=double(0)  BitMaskRealWorld=Real World Value
  Bit_XOR : simulink/Logic and Bit Operations/Bitwise Operator  logicop=XOR  UseBitMask=off  NumInputPorts=2  BitMask=double(0)  BitMaskRealWorld=Real World Value
  Bit_XOR_1 : simulink/Logic and Bit Operations/Bitwise Operator  logicop=XOR  UseBitMask=off  NumInputPorts=2  BitMask=double(0)  BitMaskRealWorld=Real World Value
  Bit_XOR_2 : simulink/Logic and Bit Operations/Bitwise Operator  logicop=XOR  UseBitMask=off  NumInputPorts=2  BitMask=double(0)  BitMaskRealWorld=Real World Value
  S : Outport  OutDataTypeStr=fixdt(0, 1, 0)  SampleTime=-1
  C : Outport  Port=2  OutDataTypeStr=fixdt(0, 1, 0)  SampleTime=-1
  wires:
  in1/1 -> Bit_XOR_2/1, Bit_AND/1, Bit_XOR_1/1
  in2/1 -> Bit_XOR_2/2, Bit_AND/2, Bit_XOR_1/2
  Cin/1 -> Bit_AND_1/1, Bit_XOR/2
  Bit_AND_1/1 -> Bit_OR/2
  Bit_OR/1 -> C/1
  Bit_XOR_2/1 -> Bit_AND_1/2
  Bit_AND/1 -> Bit_OR/1
  Bit_XOR/1 -> S/1
  Bit_XOR_1/1 -> Bit_XOR/1

== system run_small_function_cov_bitadder/For Iterator Subsystem/train_top/batch/train_sub/conv_sig/filter dim iter /i ietar Subsystem/Subsystem/For Iterator Subsystem/mac/wt_multi/ra/fa17 ==
  in1 : Inport  OutDataTypeStr=fixdt(0, 1, 0)  SampleTime=-1
  in2 : Inport  Port=2  OutDataTypeStr=fixdt(0, 1, 0)  SampleTime=-1
  Cin : Inport  Port=3  OutDataTypeStr=fixdt(0, 1, 0)  SampleTime=-1
  Bit_AND : simulink/Logic and Bit Operations/Bitwise Operator  logicop=AND  UseBitMask=off  NumInputPorts=2  BitMask=double(0)  BitMaskRealWorld=Real World Value
  Bit_AND_1 : simulink/Logic and Bit Operations/Bitwise Operator  logicop=AND  UseBitMask=off  NumInputPorts=2  BitMask=double(0)  BitMaskRealWorld=Real World Value
  Bit_OR : simulink/Logic and Bit Operations/Bitwise Operator  logicop=OR  UseBitMask=off  NumInputPorts=2  BitMask=double(0)  BitMaskRealWorld=Real World Value
  Bit_XOR : simulink/Logic and Bit Operations/Bitwise Operator  logicop=XOR  UseBitMask=off  NumInputPorts=2  BitMask=double(0)  BitMaskRealWorld=Real World Value
  Bit_XOR_1 : simulink/Logic and Bit Operations/Bitwise Operator  logicop=XOR  UseBitMask=off  NumInputPorts=2  BitMask=double(0)  BitMaskRealWorld=Real World Value
  Bit_XOR_2 : simulink/Logic and Bit Operations/Bitwise Operator  logicop=XOR  UseBitMask=off  NumInputPorts=2  BitMask=double(0)  BitMaskRealWorld=Real World Value
  S : Outport  OutDataTypeStr=fixdt(0, 1, 0)  SampleTime=-1
  C : Outport  Port=2  OutDataTypeStr=fixdt(0, 1, 0)  SampleTime=-1
  wires:
  in1/1 -> Bit_XOR_2/1, Bit_AND/1, Bit_XOR_1/1
  Bit_AND_1/1 -> Bit_OR/2
  Bit_XOR_1/1 -> Bit_XOR/1
  Bit_OR/1 -> C/1
  Cin/1 -> Bit_AND_1/1, Bit_XOR/2
  Bit_XOR_2/1 -> Bit_AND_1/2
  in2/1 -> Bit_XOR_2/2, Bit_AND/2, Bit_XOR_1/2
  Bit_XOR/1 -> S/1
  Bit_AND/1 -> Bit_OR/1

== system run_small_function_cov_bitadder/For Iterator Subsystem/train_top/batch/train_sub/conv_sig/filter dim iter /i ietar Subsystem/Subsystem/For Iterator Subsystem/mac/wt_multi/ra/fa18 ==
  in1 : Inport  OutDataTypeStr=fixdt(0, 1, 0)  SampleTime=-1
  in2 : Inport  Port=2  OutDataTypeStr=fixdt(0, 1, 0)  SampleTime=-1
  Cin : Inport  Port=3  OutDataTypeStr=fixdt(0, 1, 0)  SampleTime=-1
  Bit_AND : simulink/Logic and Bit Operations/Bitwise Operator  logicop=AND  UseBitMask=off  NumInputPorts=2  BitMask=double(0)  BitMaskRealWorld=Real World Value
  Bit_AND_1 : simulink/Logic and Bit Operations/Bitwise Operator  logicop=AND  UseBitMask=off  NumInputPorts=2  BitMask=double(0)  BitMaskRealWorld=Real World Value
  Bit_OR : simulink/Logic and Bit Operations/Bitwise Operator  logicop=OR  UseBitMask=off  NumInputPorts=2  BitMask=double(0)  BitMaskRealWorld=Real World Value
  Bit_XOR : simulink/Logic and Bit Operations/Bitwise Operator  logicop=XOR  UseBitMask=off  NumInputPorts=2  BitMask=double(0)  BitMaskRealWorld=Real World Value
  Bit_XOR_1 : simulink/Logic and Bit Operations/Bitwise Operator  logicop=XOR  UseBitMask=off  NumInputPorts=2  BitMask=double(0)  BitMaskRealWorld=Real World Value
  Bit_XOR_2 : simulink/Logic and Bit Operations/Bitwise Operator  logicop=XOR  UseBitMask=off  NumInputPorts=2  BitMask=double(0)  BitMaskRealWorld=Real World Value
  S : Outport  OutDataTypeStr=fixdt(0, 1, 0)  SampleTime=-1
  C : Outport  Port=2  OutDataTypeStr=fixdt(0, 1, 0)  SampleTime=-1
  wires:
  in2/1 -> Bit_XOR_2/2, Bit_AND/2, Bit_XOR_1/2
  Bit_AND_1/1 -> Bit_OR/2
  Bit_OR/1 -> C/1
  Bit_XOR/1 -> S/1
  Bit_XOR_1/1 -> Bit_XOR/1
  in1/1 -> Bit_XOR_2/1, Bit_AND/1, Bit_XOR_1/1
  Cin/1 -> Bit_AND_1/1, Bit_XOR/2
  Bit_XOR_2/1 -> Bit_AND_1/2
  Bit_AND/1 -> Bit_OR/1

== system run_small_function_cov_bitadder/For Iterator Subsystem/train_top/batch/train_sub/conv_sig/filter dim iter /i ietar Subsystem/Subsystem/For Iterator Subsystem/mac/wt_multi/ra/fa19 ==
  in1 : Inport  OutDataTypeStr=fixdt(0, 1, 0)  SampleTime=-1
  in2 : Inport  Port=2  OutDataTypeStr=fixdt(0, 1, 0)  SampleTime=-1
  Cin : Inport  Port=3  OutDataTypeStr=fixdt(0, 1, 0)  SampleTime=-1
  Bit_AND : simulink/Logic and Bit Operations/Bitwise Operator  logicop=AND  UseBitMask=off  NumInputPorts=2  BitMask=double(0)  BitMaskRealWorld=Real World Value
  Bit_AND_1 : simulink/Logic and Bit Operations/Bitwise Operator  logicop=AND  UseBitMask=off  NumInputPorts=2  BitMask=double(0)  BitMaskRealWorld=Real World Value
  Bit_OR : simulink/Logic and Bit Operations/Bitwise Operator  logicop=OR  UseBitMask=off  NumInputPorts=2  BitMask=double(0)  BitMaskRealWorld=Real World Value
  Bit_XOR : simulink/Logic and Bit Operations/Bitwise Operator  logicop=XOR  UseBitMask=off  NumInputPorts=2  BitMask=double(0)  BitMaskRealWorld=Real World Value
  Bit_XOR_1 : simulink/Logic and Bit Operations/Bitwise Operator  logicop=XOR  UseBitMask=off  NumInputPorts=2  BitMask=double(0)  BitMaskRealWorld=Real World Value
  Bit_XOR_2 : simulink/Logic and Bit Operations/Bitwise Operator  logicop=XOR  UseBitMask=off  NumInputPorts=2  BitMask=double(0)  BitMaskRealWorld=Real World Value
  S : Outport  OutDataTypeStr=fixdt(0, 1, 0)  SampleTime=-1
  C : Outport  Port=2  OutDataTypeStr=fixdt(0, 1, 0)  SampleTime=-1
  wires:
  in1/1 -> Bit_XOR_2/1, Bit_AND/1, Bit_XOR_1/1
  in2/1 -> Bit_XOR_2/2, Bit_AND/2, Bit_XOR_1/2
  Bit_AND_1/1 -> Bit_OR/2
  Bit_OR/1 -> C/1
  Bit_XOR_2/1 -> Bit_AND_1/2
  Bit_AND/1 -> Bit_OR/1
  Cin/1 -> Bit_AND_1/1, Bit_XOR/2
  Bit_XOR/1 -> S/1
  Bit_XOR_1/1 -> Bit_XOR/1

== system run_small_function_cov_bitadder/For Iterator Subsystem/train_top/batch/train_sub/conv_sig/filter dim iter /i ietar Subsystem/Subsystem/For Iterator Subsystem/mac/wt_multi/ra/fa2 ==
  in1 : Inport  OutDataTypeStr=fixdt(0, 1, 0)  SampleTime=-1
  in2 : Inport  Port=2  OutDataTypeStr=fixdt(0, 1, 0)  SampleTime=-1
  Cin : Inport  Port=3  OutDataTypeStr=fixdt(0, 1, 0)  SampleTime=-1
  Bit_AND : simulink/Logic and Bit Operations/Bitwise Operator  logicop=AND  UseBitMask=off  NumInputPorts=2  BitMask=double(0)  BitMaskRealWorld=Real World Value
  Bit_AND_1 : simulink/Logic and Bit Operations/Bitwise Operator  logicop=AND  UseBitMask=off  NumInputPorts=2  BitMask=double(0)  BitMaskRealWorld=Real World Value
  Bit_OR : simulink/Logic and Bit Operations/Bitwise Operator  logicop=OR  UseBitMask=off  NumInputPorts=2  BitMask=double(0)  BitMaskRealWorld=Real World Value
  Bit_XOR : simulink/Logic and Bit Operations/Bitwise Operator  logicop=XOR  UseBitMask=off  NumInputPorts=2  BitMask=double(0)  BitMaskRealWorld=Real World Value
  Bit_XOR_1 : simulink/Logic and Bit Operations/Bitwise Operator  logicop=XOR  UseBitMask=off  NumInputPorts=2  BitMask=double(0)  BitMaskRealWorld=Real World Value
  Bit_XOR_2 : simulink/Logic and Bit Operations/Bitwise Operator  logicop=XOR  UseBitMask=off  NumInputPorts=2  BitMask=double(0)  BitMaskRealWorld=Real World Value
  S : Outport  OutDataTypeStr=fixdt(0, 1, 0)  SampleTime=-1
  C : Outport  Port=2  OutDataTypeStr=fixdt(0, 1, 0)  SampleTime=-1
  wires:
  in1/1 -> Bit_XOR_2/1, Bit_AND/1, Bit_XOR_1/1
  in2/1 -> Bit_XOR_2/2, Bit_AND/2, Bit_XOR_1/2
  Cin/1 -> Bit_AND_1/1, Bit_XOR/2
  Bit_AND_1/1 -> Bit_OR/2
  Bit_OR/1 -> C/1
  Bit_XOR/1 -> S/1
  Bit_XOR_2/1 -> Bit_AND_1/2
  Bit_XOR_1/1 -> Bit_XOR/1
  Bit_AND/1 -> Bit_OR/1

== system run_small_function_cov_bitadder/For Iterator Subsystem/train_top/batch/train_sub/conv_sig/filter dim iter /i ietar Subsystem/Subsystem/For Iterator Subsystem/mac/wt_multi/ra/fa20 ==
  in1 : Inport  OutDataTypeStr=fixdt(0, 1, 0)  SampleTime=-1
  in2 : Inport  Port=2  OutDataTypeStr=fixdt(0, 1, 0)  SampleTime=-1
  Cin : Inport  Port=3  OutDataTypeStr=fixdt(0, 1, 0)  SampleTime=-1
  Bit_AND : simulink/Logic and Bit Operations/Bitwise Operator  logicop=AND  UseBitMask=off  NumInputPorts=2  BitMask=double(0)  BitMaskRealWorld=Real World Value
  Bit_AND_1 : simulink/Logic and Bit Operations/Bitwise Operator  logicop=AND  UseBitMask=off  NumInputPorts=2  BitMask=double(0)  BitMaskRealWorld=Real World Value
  Bit_OR : simulink/Logic and Bit Operations/Bitwise Operator  logicop=OR  UseBitMask=off  NumInputPorts=2  BitMask=double(0)  BitMaskRealWorld=Real World Value
  Bit_XOR : simulink/Logic and Bit Operations/Bitwise Operator  logicop=XOR  UseBitMask=off  NumInputPorts=2  BitMask=double(0)  BitMaskRealWorld=Real World Value
  Bit_XOR_1 : simulink/Logic and Bit Operations/Bitwise Operator  logicop=XOR  UseBitMask=off  NumInputPorts=2  BitMask=double(0)  BitMaskRealWorld=Real World Value
  Bit_XOR_2 : simulink/Logic and Bit Operations/Bitwise Operator  logicop=XOR  UseBitMask=off  NumInputPorts=2  BitMask=double(0)  BitMaskRealWorld=Real World Value
  S : Outport  OutDataTypeStr=fixdt(0, 1, 0)  SampleTime=-1
  C : Outport  Port=2  OutDataTypeStr=fixdt(0, 1, 0)  SampleTime=-1
  wires:
  in2/1 -> Bit_XOR_2/2, Bit_AND/2, Bit_XOR_1/2
  Cin/1 -> Bit_AND_1/1, Bit_XOR/2
  Bit_AND_1/1 -> Bit_OR/2
  in1/1 -> Bit_XOR_2/1, Bit_AND/1, Bit_XOR_1/1
  Bit_OR/1 -> C/1
  Bit_AND/1 -> Bit_OR/1
  Bit_XOR_2/1 -> Bit_AND_1/2
  Bit_XOR/1 -> S/1
  Bit_XOR_1/1 -> Bit_XOR/1
